simulink model "mp"  (R2023a)
settings: Solver=VariableStepAuto  StartTime=0.0  StopTime=0.5  RelTol=1e-3
undefined symbols (not defined in the file): Ion, Lithium
libraries: spsBreakerLib x3, spsBatteryLib x1, spsCurrentMeasurementLib x1, spsDCVoltageSourceLib x1, spsPVArrayLib x1, spsSeriesRLCBranchLib x1, spsVoltageMeasurementLib x1, sps_lib x1
settings Model: Creator=kumar  LastModifiedBy=kumar

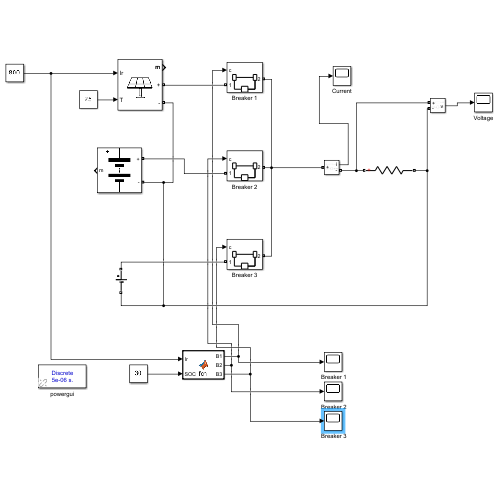
[thumbnail: Simulink's stored preview of the top-level diagram]
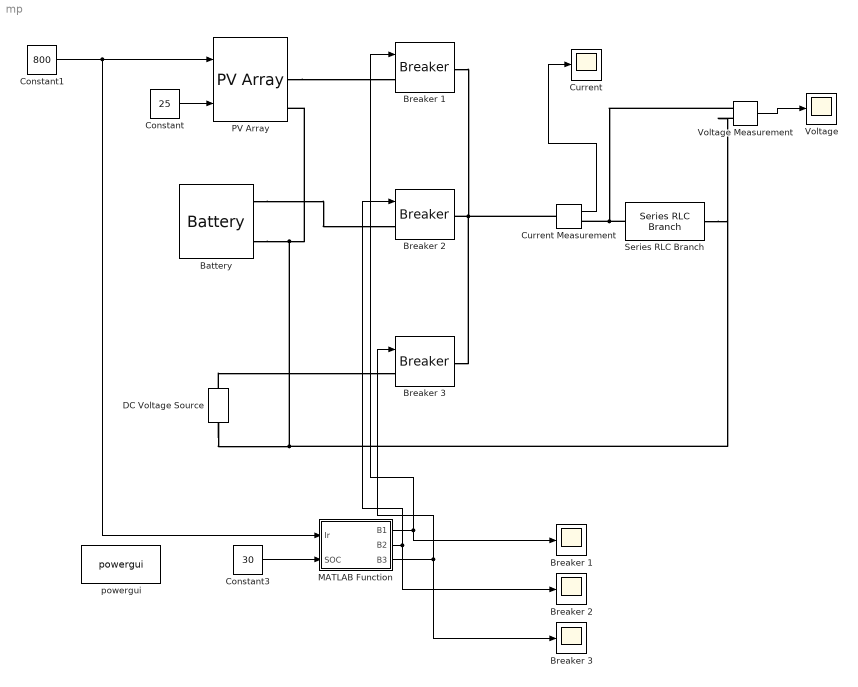
== system mp ==
  " Breaker 1" : Scope
  " Breaker 2" : Scope
  " Breaker 3" : Scope
  Battery : spsBatteryLib/Battery  BatType=Lithium-Ion  ShowTempParam=off  ThermalPreset=no  ShowAgeParam=off  NomV=240  NomQ=50  SOC=80  Batt_Tr=30  PresetModel=on  MaxQ=50  MinV=180  FullV=279.3569  Dis_rate=21.7391  R=0.048  Normal_OP=45.2174  expZone="[259.2926      2.456522]"  current=[6.5 13 32.5]  Units=Time  Tci=20  NomT=20  T2=-30  MaxQ2=4.8  FullV2=7.1  Normal_OP2=5.655  expZone2="[6.58           1]"  Rca=0.6  ti=2000  Dp=0  Neq0=0  Tsim=1e6  Ta1=25  Qeol=5.4*0.9  Reol=0.013333*1.2  Char_age=[2.3478, 3]  Dis_age=[2.3478, 10]  N1=1500  N2=10500  N3=1000  N4=1400  Ta2=45  N5=950
  Breaker 1 : spsBreakerLib/Breaker  InitialState=1  SwitchingTimes="[1/60  5/60]"  External=on  BreakerResistance=0.01  SnubberResistance=1e6  SnubberCapacitance=inf  Measurements=None  MoreParameters=on  NoBreakLoop=off
  Breaker 2 : spsBreakerLib/Breaker  InitialState=1  SwitchingTimes="[1/60  5/60]"  External=on  BreakerResistance=0.01  SnubberResistance=1e6  SnubberCapacitance=inf  Measurements=None  MoreParameters=on  NoBreakLoop=off
  Breaker 3 : spsBreakerLib/Breaker  InitialState=1  SwitchingTimes="[1/60  5/60]"  External=on  BreakerResistance=0.01  SnubberResistance=1e6  SnubberCapacitance=inf  Measurements=None  MoreParameters=on  NoBreakLoop=off
  Constant : Constant  Value=25
  Constant1 : Constant  Value=800
  Constant3 : Constant  Value=30
  Current : Scope
  Current Measurement : spsCurrentMeasurementLib/Current Measurement  PhasorSimulation=off  OutputType=Complex  PSBequivalent=0
  DC Voltage Source : spsDCVoltageSourceLib/DC Voltage Source  Amplitude=240  Measurements=None
  MATLAB Function : MATLAB Function  TreatAsAtomicUnit=on
  PV Array : spsPVArrayLib/PV Array  Npar=1  Nser=10  PlotType=array @ 1000 W/m2 & specified temperatures  S_vec="[ 1000  500  100 ]"  Temp_C_vec="[ 45 25  ]"  ModuleName=User-defined  PlotWhenSelected=off  Pm=213.15  Ncell=60  Voc=36.3  Isc=7.84  Vm=29  Im=7.35  beta_Voc_pc=-0.36099  alpha_Isc_pc=0.102  beta_Voc=-0.13104  alpha_Isc=0.0079968  IL=7.8654  I0=2.9273e-10  nI=0.98119  Rsh=313.0553  Rs=0.39381  RobustModel=off  RobustCellTemperature=313.3991  BAL=on  Tc=1e-6  Tfilter=5e-5
  Series RLC Branch : spsSeriesRLCBranchLib/Series RLC Branch  LConnTagsString=__new0  RConnTagsString=__new0  BranchType=R  Resistance=20  Inductance=1e-3  SetiL0=off  InitialCurrent=0  Capacitance=1e-6  Setx0=off  InitialVoltage=0  Measurements=None
  Voltage : Scope
  Voltage Measurement : spsVoltageMeasurementLib/Voltage Measurement  PhasorSimulation=off  OutputType=Complex  PSBequivalent=0
  powergui : sps_lib/powergui  Priority=1  SimulationMode=Discrete  SampleTime=5e-6  frequency=60  Iterations=50  frequencyindice=0  Pbase=100e6  ErrMax=1e-4  UnitsV=kV  UnitsW=MW  buscounter=0  FunctionMessages=off  echomessages=off  EnableUseOfTLC=off  CurrentSourceSwitches=off  DisableSnubberDevices=off  DisableRonSwitches=off  DisableVfSwitches=off  DisplayEquations=off  AutomaticDiscreteSolvers=off  SolverType=Tustin/Backward Euler (TBE)  Interpol=off  ExternalGateDelay=off  methode=off  Ts=100  x0status=blocks  SPID=on  SwTol=0  HookPort=off  NonlinearTolerance=1e-4  nMaxIteration=100  ContinueOnMaxIteration=off  RestoreLinks=warning  ResistiveCurrentMeasurement=off  Frange=[0:2:500]  Ylog=off  Xlog=on  ShowGrid=off  save=off  variable=ZData  structure=0  ZoomFFT=off  StartTime=0.0  cycles=1  DisplayStyle=1  fundamental=60  FreqAxis=off  MaxFrequency=1000  frequencyindicesteady=1  RmsSteady=1  display=off
  wires:
  Constant/1 -> PV Array/2
  Constant1/1 -> MATLAB Function/1(Ir), PV Array/1
  Constant3/1 -> MATLAB Function/2(SOC)
  MATLAB Function/1(B1) -> " Breaker 1"/1, Breaker 1/1
  MATLAB Function/2(B2) -> " Breaker 2"/1, Breaker 2/1
  MATLAB Function/3(B3) -> " Breaker 3"/1, Breaker 3/1
  Voltage Measurement/1 -> Voltage/1
  Current Measurement/1 -> Current/1
  connections:
  PV Array/RConn1 -- Breaker 1/LConn1
  DC Voltage Source/RConn1 -- Breaker 3/LConn1
  Battery/LConn1 -- Breaker 2/LConn1
  Breaker 1/RConn1 -- Current Measurement/LConn1 -- Breaker 3/RConn1 -- Breaker 2/RConn1
  Series RLC Branch/LConn1 -- Voltage Measurement/LConn1 -- Current Measurement/RConn1
  Battery/LConn2 -- Voltage Measurement/LConn2 -- Series RLC Branch/RConn1 -- DC Voltage Source/LConn1 -- PV Array/RConn2

== matlab function mp/MATLAB Function ==
  data: Ir input; B1 output; SOC input; B2 output; B3 output
function [B1, B2, B3] = fcn(Ir, SOC)
if Ir > 800
    B1 = 1;  % PV ON
    B2 = 0;
    B3 = 0;

elseif SOC > 30
    B1 = 0;
    B2 = 1;  % Battery ON
    B3 = 0;

else
    B1 = 0;
    B2 = 0;
    B3 = 1;  % Backup ON
end
